simulink model "block_test"  (R2022b)
settings: Solver=VariableStepAuto  StartTime=0.0  StopTime=10.0  RelTol=1e-3
settings Model: Creator=phatdo  LastModifiedBy=phatdo

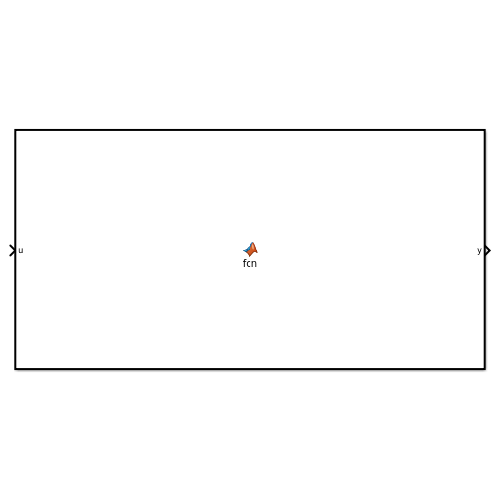
[thumbnail: Simulink's stored preview of the top-level diagram]
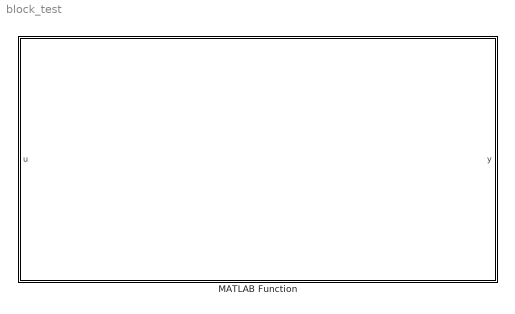
== system block_test ==
  MATLAB Function : MATLAB Function  TreatAsAtomicUnit=on

== matlab function block_test/MATLAB Function ==
  data: u input; y output
function y = fcn(u)

y = u;
